simulink model "IEEE30_case"  (R2024b)
settings: Solver=FixedStepAuto  StartTime=0  StopTime=5  FixedStep=1e-7  RelTol=1e-3
values from neighbouring files (symbols this model uses):
  GFL_DFIG_7_C_bus = 0.08    [IEEE30_case_parameters.m]
  GFL_DFIG_7_D_mutual = 2.500000e+3    (= 2500)    [IEEE30_case_parameters.m]
  GFL_DFIG_7_f0 = 60    [IEEE30_case_parameters.m]
  GFL_DFIG_7_gPLLi = 3200    [IEEE30_case_parameters.m]
  GFL_DFIG_7_gPLLp = 650    [IEEE30_case_parameters.m]
  GFL_DFIG_7_H_WT = 0.4    [IEEE30_case_parameters.m]
  GFL_DFIG_7_Hg = 0.8    [IEEE30_case_parameters.m]
  GFL_DFIG_7_Igq_ref = 0    [IEEE30_case_parameters.m]
  GFL_DFIG_7_Ird_ref = 704.45696    [IEEE30_case_parameters.m]
  GFL_DFIG_7_KI_V = -300000    [IEEE30_case_parameters.m]
  GFL_DFIG_7_KP_V = -1000    [IEEE30_case_parameters.m]
  GFL_DFIG_7_Ksh = 1.254300e+4    (= 12543)    [IEEE30_case_parameters.m]
  GFL_DFIG_7_Lg = 0.000483    [IEEE30_case_parameters.m]
  GFL_DFIG_7_Lm_pu = 4    [IEEE30_case_parameters.m]
  GFL_DFIG_7_N = 100    [IEEE30_case_parameters.m]
  GFL_DFIG_7_p = 2    [IEEE30_case_parameters.m]
  GFL_DFIG_7_Pitch = 0    [IEEE30_case_parameters.m]
  GFL_DFIG_7_R = 44    [IEEE30_case_parameters.m]
  GFL_DFIG_7_Rg = 2.000000e-5    (= 2e-05)    [IEEE30_case_parameters.m]
  GFL_DFIG_7_rho = 1.225    [IEEE30_case_parameters.m]
  GFL_DFIG_7_rPLLi = 4500    [IEEE30_case_parameters.m]
  GFL_DFIG_7_rPLLp = 620    [IEEE30_case_parameters.m]
  GFL_DFIG_7_Rs_pu = 0.011    [IEEE30_case_parameters.m]
  GFL_DFIG_7_Sbase = 2.000000e+6    (= 2000000)    [IEEE30_case_parameters.m]
  GFL_DFIG_7_ugq_ref = 0    [IEEE30_case_parameters.m]
  GFL_DFIG_7_usd_ref = 0    [IEEE30_case_parameters.m]
  GFL_DFIG_7_Vbase = 690    [IEEE30_case_parameters.m]
  GFL_DFIG_7_Vdc_ref = 1200    [IEEE30_case_parameters.m]
  GFL_DFIG_7_wind = 12    [IEEE30_case_parameters.m]
  GFL_DFIG_7_wm_ref = 518.184209    [IEEE30_case_parameters.m]
  SG_D_13_D = 0.01056    [IEEE30_case_parameters.m]
  SG_D_13_EnableSaturation = 0    [IEEE30_case_parameters.m]
  SG_D_13_f0 = 60    [IEEE30_case_parameters.m]
  SG_D_13_H = 7.5    [IEEE30_case_parameters.m]
  SG_D_13_K_A = 20    [IEEE30_case_parameters.m]
  SG_D_13_K_E = 1.000000e+1    (= 10)    [IEEE30_case_parameters.m]
  SG_D_13_K_F = 2.363    [IEEE30_case_parameters.m]
  SG_D_13_K_s = 0.5    [IEEE30_case_parameters.m]
  SG_D_13_R_a = 0.001088    [IEEE30_case_parameters.m]
  SG_D_13_S_A = 1    [IEEE30_case_parameters.m]
  SG_D_13_S_B = 0.103    [IEEE30_case_parameters.m]
  SG_D_13_S_N = 10.659857    [IEEE30_case_parameters.m]
  SG_D_13_SpeedPara = 200    [IEEE30_case_parameters.m]
  SG_D_13_T_0 = 0.370163    [IEEE30_case_parameters.m]
  SG_D_13_T_1 = 0.3    [IEEE30_case_parameters.m]
  SG_D_13_T_2 = 0.05    [IEEE30_case_parameters.m]
  SG_D_13_T_3 = 0.02    [IEEE30_case_parameters.m]
  SG_D_13_T_4 = 0.005    [IEEE30_case_parameters.m]
  SG_D_13_T_A = 0.02    [IEEE30_case_parameters.m]
  SG_D_13_T_dd = 8.000000e+0    (= 8)    [IEEE30_case_parameters.m]
  SG_D_13_T_ddd = 0.04    [IEEE30_case_parameters.m]
  SG_D_13_T_E = 0.314    [IEEE30_case_parameters.m]
  SG_D_13_T_F = 0.35    [IEEE30_case_parameters.m]
  SG_D_13_T_qd = 0.8    [IEEE30_case_parameters.m]
  SG_D_13_T_qdd = 0.02    [IEEE30_case_parameters.m]
  SG_D_13_T_speed = 0.1    [IEEE30_case_parameters.m]
  SG_D_13_T_w = 0.5    [IEEE30_case_parameters.m]
  SG_D_13_V_ref = 1.696619    [IEEE30_case_parameters.m]
  SG_D_13_w_ref = 376.991118    [IEEE30_case_parameters.m]
  SG_D_13_x_d = 1.9    [IEEE30_case_parameters.m]
  SG_D_13_x_dd = 0.302    [IEEE30_case_parameters.m]
  SG_D_13_x_ddd = 0.204    [IEEE30_case_parameters.m]
  SG_D_13_x_l = 0.05    [IEEE30_case_parameters.m]
  SG_D_13_x_q = 1.3    [IEEE30_case_parameters.m]
  SG_D_13_x_qd = 0.5    [IEEE30_case_parameters.m]
  SG_D_13_x_qdd = 0.3    [IEEE30_case_parameters.m]
  SG_D_1_D = 0.01056    [IEEE30_case_parameters.m]
  SG_D_1_EnableSaturation = 0    [IEEE30_case_parameters.m]
  SG_D_1_f0 = 60    [IEEE30_case_parameters.m]
  SG_D_1_H = 7.5    [IEEE30_case_parameters.m]
  SG_D_1_K_A = 20    [IEEE30_case_parameters.m]
  SG_D_1_K_E = 1.000000e+1    (= 10)    [IEEE30_case_parameters.m]
  SG_D_1_K_F = 2.363    [IEEE30_case_parameters.m]
  SG_D_1_K_s = 0.5    [IEEE30_case_parameters.m]
  SG_D_1_R_a = 0.001088    [IEEE30_case_parameters.m]
  SG_D_1_S_A = 1    [IEEE30_case_parameters.m]
  SG_D_1_S_B = 0.103    [IEEE30_case_parameters.m]
  SG_D_1_S_N = 10.659857    [IEEE30_case_parameters.m]
  SG_D_1_SpeedPara = 200    [IEEE30_case_parameters.m]
  SG_D_1_T_0 = 0.259812    [IEEE30_case_parameters.m]
  SG_D_1_T_1 = 0.3    [IEEE30_case_parameters.m]
  SG_D_1_T_2 = 0.05    [IEEE30_case_parameters.m]
  SG_D_1_T_3 = 0.02    [IEEE30_case_parameters.m]
  SG_D_1_T_4 = 0.005    [IEEE30_case_parameters.m]
  SG_D_1_T_A = 0.02    [IEEE30_case_parameters.m]
  SG_D_1_T_dd = 8.000000e+0    (= 8)    [IEEE30_case_parameters.m]
  SG_D_1_T_ddd = 0.04    [IEEE30_case_parameters.m]
  SG_D_1_T_E = 0.314    [IEEE30_case_parameters.m]
  SG_D_1_T_F = 0.35    [IEEE30_case_parameters.m]
  SG_D_1_T_qd = 0.8    [IEEE30_case_parameters.m]
  SG_D_1_T_qdd = 0.02    [IEEE30_case_parameters.m]
  SG_D_1_T_speed = 0.1    [IEEE30_case_parameters.m]
  SG_D_1_T_w = 0.5    [IEEE30_case_parameters.m]
  SG_D_1_V_ref = 1.544107    [IEEE30_case_parameters.m]
  SG_D_1_w_ref = 376.991118    [IEEE30_case_parameters.m]
  SG_D_1_x_d = 1.9    [IEEE30_case_parameters.m]
  SG_D_1_x_dd = 0.302    [IEEE30_case_parameters.m]
  SG_D_1_x_ddd = 0.204    [IEEE30_case_parameters.m]
  SG_D_1_x_l = 0.05    [IEEE30_case_parameters.m]
  SG_D_1_x_q = 1.3    [IEEE30_case_parameters.m]
  SG_D_1_x_qd = 0.5    [IEEE30_case_parameters.m]
  SG_D_1_x_qdd = 0.3    [IEEE30_case_parameters.m]
  SG_D_22_D = 0.01056    [IEEE30_case_parameters.m]
  SG_D_22_EnableSaturation = 0    [IEEE30_case_parameters.m]
  SG_D_22_f0 = 60    [IEEE30_case_parameters.m]
  SG_D_22_H = 7.5    [IEEE30_case_parameters.m]
  SG_D_22_K_A = 20    [IEEE30_case_parameters.m]
  SG_D_22_K_E = 1.000000e+1    (= 10)    [IEEE30_case_parameters.m]
  SG_D_22_K_F = 2.363    [IEEE30_case_parameters.m]
  SG_D_22_K_s = 0.5    [IEEE30_case_parameters.m]
  SG_D_22_R_a = 0.001088    [IEEE30_case_parameters.m]
  SG_D_22_S_A = 1    [IEEE30_case_parameters.m]
  SG_D_22_S_B = 0.103    [IEEE30_case_parameters.m]
  SG_D_22_S_N = 10.659857    [IEEE30_case_parameters.m]
  SG_D_22_SpeedPara = 200    [IEEE30_case_parameters.m]
  SG_D_22_T_0 = 0.216121    [IEEE30_case_parameters.m]
  SG_D_22_T_1 = 0.3    [IEEE30_case_parameters.m]
  SG_D_22_T_2 = 0.05    [IEEE30_case_parameters.m]
  SG_D_22_T_3 = 0.02    [IEEE30_case_parameters.m]
  SG_D_22_T_4 = 0.005    [IEEE30_case_parameters.m]
  ... (+126 more)
(part 24 of 27)

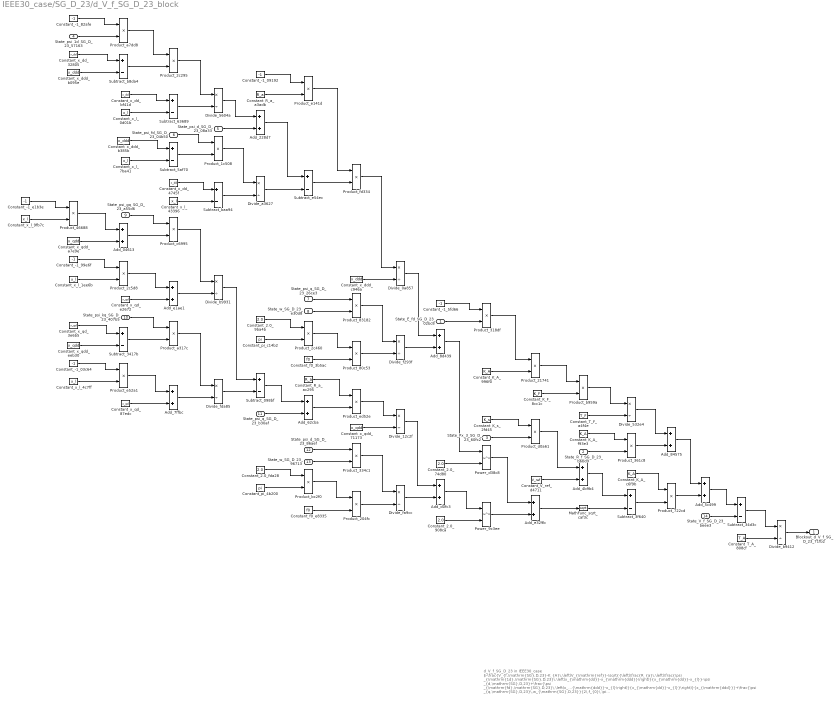
== system IEEE30_case/SG_D_23/d_V_f_SG_D_23_block ==
  note: d_V_f_SG_D_23 in IEEE30_case
      | $-\frac{V_{f,\mathrm{SG},D,23}-K_{A}\,\left(V_{\mathrm{ref}}-\sqrt{{\left(\frac{R_{a}\,\left(\frac{\psi _{\mathrm{1d},\mathrm{SG},D,23}\,\left(x_{\mathrm{dd}}-x_{\mathrm{ddd}}\right)}{x_{\mathrm{dd}}-x_{l}}-\psi _{d,\mathrm{SG},D,23}+\frac{\psi _{\mathrm{fd},\mathrm{SG},D,23}\,\left(x_{\mathrm{ddd}}-x_{l}\right)}{x_{\mathrm{dd}}-x_{l}}\right)}{x_{\mathrm{ddd}}}+\frac{\psi _{q,\mathrm{SG},D,23}\,w_{\mathrm{SG},D,23}}{2\,f_{0}\,\pi }\right)}^2+{\left(\frac{R_{a}\,\left(\psi _{q,\mathrm{SG},D,23}+\frac{\psi _{\mathrm{gq},\mathrm{SG},D,23}\,\left(x_{l}-x_{\mathrm{qdd}}\right)}{x_{l}-x_{\mathrm{qd}}}+\frac{\psi _{\mathrm{kq},\mathrm{SG},D,23}\,\left(x_{\mathrm{qd}}-x_{\mathrm{qdd}}\right)}{x_{l}-x_{\mathrm{qd}}}\right)}{x_{\mathrm{qdd}}}+\frac{\psi _{d,\mathrm{SG},D,23}\,w_{\mathrm{SG},D,23}}{2\,f_{0}\,\pi }\right)}^2}+K_{s}\,\mathrm{Px}_{3,\mathrm{SG},D,23}\right)-K_{A}\,R_{f,\mathrm{SG},D,23}+\frac{E_{\mathrm{fd},\mathrm{SG},D,23}\,K_{A}\,K_{F}}{T_{F}}}{T_{A}}$
      | Automatically generated on 2025-11-01 18:37:37 .
  State_E_fd_SG_D_23_02bc8 : Inport
  State_R_f_SG_D_23_b6bd9 : Inport  Port=2
  State_Px_3_SG_D_23_60fc2 : Inport  Port=3
  State_psi_1d_SG_D_23_57163 : Inport  Port=4
  State_psi_d_SG_D_23_08a33 : Inport  Port=5
  State_psi_fd_SG_D_23_04b50 : Inport  Port=6
  State_psi_q_SG_D_23_26ce3 : Inport  Port=7
  State_w_SG_D_23_e30d8 : Inport  Port=8
  State_psi_gq_SG_D_23_a55d6 : Inport  Port=9
  State_psi_kq_SG_D_23_407b5 : Inport  Port=10
  State_psi_q_SG_D_23_b30af : Inport  Port=11
  State_psi_d_SG_D_23_86aef : Inport  Port=12
  State_w_SG_D_23_96713 : Inport  Port=13
  State_V_f_SG_D_23_beee3 : Inport  Port=14
  Add_04613 : Sum
  Add_228d7 : Sum
  Add_4b9b4 : Sum
  Add_5c499 : Sum
  Add_62cba : Sum
  Add_7ffbc : Sum
  Add_84575 : Sum
  Add_8d439 : Sum
  Add_d0fc3 : Sum
  Add_e1ae1 : Sum
  Add_e329b : Sum
  Constant_-1_03c64 : Constant  Value=-1
  Constant_-1_09192 : Constant  Value=-1
  Constant_-1_5fd66 : Constant  Value=-1
  Constant_-1_82afe : Constant  Value=-1
  Constant_-1_99e6f : Constant  Value=-1
  Constant_-1_e1b3e : Constant  Value=-1
  Constant_2.0_74d80 : Constant  Value=2.0
  Constant_2.0_908ca : Constant  Value=2.0
  Constant_2.0_9ba4b : Constant  Value=2.0
  Constant_2.0_fda28 : Constant  Value=2.0
  Constant_K_A_996f0 : Constant  Value=K_A
  Constant_K_A_c6f9b : Constant  Value=K_A
  Constant_K_A_f93e3 : Constant  Value=K_A
  Constant_K_F_8cc1c : Constant  Value=K_F
  Constant_K_s_2fd45 : Constant  Value=K_s
  Constant_R_a_a3adb : Constant  Value=R_a
  Constant_R_a_ac295 : Constant  Value=R_a
  Constant_T_A_808cf : Constant  Value=T_A
  Constant_T_F_a4f4e : Constant  Value=T_F
  Constant_V_ref_d4711 : Constant  Value=V_ref
  Constant_f0_3b5ac : Constant  Value=f0
  Constant_f0_e8335 : Constant  Value=f0
  Constant_pi_4b200 : Constant  Value=pi
  Constant_pi_c14b2 : Constant  Value=pi
  Constant_x_dd_32805 : Constant  Value=x_dd
  Constant_x_dd_4745f : Constant  Value=x_dd
  Constant_x_dd_bf41d : Constant  Value=x_dd
  Constant_x_ddd_b095e : Constant  Value=x_ddd
  Constant_x_ddd_b385b : Constant  Value=x_ddd
  Constant_x_ddd_c946a : Constant  Value=x_ddd
  Constant_x_l_0d01b : Constant  Value=x_l
  Constant_x_l_1ee6b : Constant  Value=x_l
  Constant_x_l_43396 : Constant  Value=x_l
  Constant_x_l_4c7ff : Constant  Value=x_l
  Constant_x_l_7ba41 : Constant  Value=x_l
  Constant_x_l_9fb7c : Constant  Value=x_l
  Constant_x_qd_3e6b5 : Constant  Value=x_qd
  Constant_x_qd_87edc : Constant  Value=x_qd
  Constant_x_qd_e2672 : Constant  Value=x_qd
  Constant_x_qdd_71173 : Constant  Value=x_qdd
  Constant_x_qdd_a7e9e : Constant  Value=x_qdd
  Constant_x_qdd_eeb30 : Constant  Value=x_qdd
  Divide_0a857 : Product  Inputs=*/
  Divide_12c2f : Product  Inputs=*/
  Divide_532e4 : Product  Inputs=*/
  Divide_5604a : Product  Inputs=*/
  Divide_a3627 : Product  Inputs=*/
  Divide_b9412 : Product  Inputs=*/
  Divide_b9931 : Product  Inputs=*/
  Divide_f293f : Product  Inputs=*/
  Divide_fa9cc : Product  Inputs=*/
  Divide_fda85 : Product  Inputs=*/
  MathFunc_sqrt_caf3c : Sqrt
  Power_9c3ee : Math  Operator=pow
  Power_d38c8 : Math  Operator=pow
  Product_1c508 : Product
  Product_204fc : Product
  Product_21741 : Product
  Product_2c295 : Product
  Product_2c460 : Product
  Product_2c5d8 : Product
  Product_318df : Product
  Product_334c1 : Product
  Product_361c8 : Product
  Product_46688 : Product
  Product_722cd : Product
  Product_80c53 : Product
  Product_83182 : Product
  Product_a317c : Product
  Product_a7dd8 : Product
  Product_b959a : Product
  Product_bc2f0 : Product
  Product_c6995 : Product
  Product_d0a61 : Product
  Product_e141d : Product
  Product_e52a1 : Product
  Product_ed52e : Product
  Product_fd334 : Product
  Subtract_098bf : Sum  Inputs=+-
  Subtract_3417b : Sum  Inputs=+-
  Subtract_34d3c : Sum  Inputs=+-
  Subtract_3f640 : Sum  Inputs=+-
  Subtract_5af70 : Sum  Inputs=+-
  Subtract_63689 : Sum  Inputs=+-
  Subtract_b8da4 : Sum  Inputs=+-
  Subtract_baa94 : Sum  Inputs=+-
  Subtract_e54ec : Sum  Inputs=+-
  Blockout_d_V_f_SG_D_23_71fb2 : Outport
  wires:
  Constant_-1_e1b3e/1 -> Product_46688/1
  Add_228d7/1 -> Subtract_e54ec/1
  Constant_x_l_9fb7c/1 -> Product_46688/2
  Constant_-1_82afe/1 -> Product_a7dd8/1
  Product_2c5d8/1 -> Add_e1ae1/1
  State_psi_1d_SG_D_23_57163/1 -> Product_a7dd8/2
  Constant_x_dd_32805/1 -> Subtract_b8da4/1
  Divide_5604a/1 -> Add_228d7/1
  Constant_x_qdd_a7e9e/1 -> Add_04613/2
  Subtract_3417b/1 -> Product_a317c/2
  Constant_x_ddd_b095e/1 -> Subtract_b8da4/2
  Product_46688/1 -> Add_04613/1
  Constant_-1_99e6f/1 -> Product_2c5d8/1
  State_psi_d_SG_D_23_86aef/1 -> Product_334c1/1
  Constant_x_l_1ee6b/1 -> Product_2c5d8/2
  State_psi_d_SG_D_23_08a33/1 -> Add_228d7/2
  Divide_0a857/1 -> Add_8d439/1
  Constant_x_qd_3e6b5/1 -> Subtract_3417b/1
  Constant_x_qdd_eeb30/1 -> Subtract_3417b/2
  Constant_-1_03c64/1 -> Product_e52a1/1
  Constant_x_l_4c7ff/1 -> Product_e52a1/2
  Constant_R_a_a3adb/1 -> Product_e141d/2
  Product_a7dd8/1 -> Product_2c295/1
  Subtract_b8da4/1 -> Product_2c295/2
  Constant_2.0_fda28/1 -> Product_bc2f0/1
  Constant_x_dd_bf41d/1 -> Subtract_63689/1
  Product_e141d/1 -> Product_fd334/1
  Add_7ffbc/1 -> Divide_fda85/2
  Constant_pi_4b200/1 -> Product_bc2f0/2
  Constant_x_l_0d01b/1 -> Subtract_63689/2
  Constant_f0_3b5ac/1 -> Product_80c53/2
  Constant_x_ddd_b385b/1 -> Subtract_5af70/1
  Constant_x_l_7ba41/1 -> Subtract_5af70/2
  State_psi_gq_SG_D_23_a55d6/1 -> Product_c6995/1
  Constant_K_A_f93e3/1 -> Product_361c8/1
  State_w_SG_D_23_e30d8/1 -> Product_83182/2
  Add_04613/1 -> Product_c6995/2
  Product_2c295/1 -> Divide_5604a/1
  Constant_x_qd_e2672/1 -> Add_e1ae1/2
  State_w_SG_D_23_96713/1 -> Product_334c1/2
  State_psi_kq_SG_D_23_407b5/1 -> Product_a317c/1
  Constant_-1_09192/1 -> Product_e141d/1
  Constant_f0_e8335/1 -> Product_204fc/2
  Product_e52a1/1 -> Add_7ffbc/1
  Constant_x_qd_87edc/1 -> Add_7ffbc/2
  Add_e1ae1/1 -> Divide_b9931/2
  Subtract_63689/1 -> Divide_5604a/2
  State_psi_fd_SG_D_23_04b50/1 -> Product_1c508/1
  Constant_pi_c14b2/1 -> Product_2c460/2
  Subtract_5af70/1 -> Product_1c508/2
  Constant_x_dd_4745f/1 -> Subtract_baa94/1
  Constant_x_l_43396/1 -> Subtract_baa94/2
  Product_c6995/1 -> Divide_b9931/1
  Product_a317c/1 -> Divide_fda85/1
  Product_1c508/1 -> Divide_a3627/1
  Subtract_baa94/1 -> Divide_a3627/2
  Divide_b9931/1 -> Subtract_098bf/1
  Divide_fda85/1 -> Subtract_098bf/2
  Divide_a3627/1 -> Subtract_e54ec/2
  Constant_2.0_9ba4b/1 -> Product_2c460/1
  Subtract_098bf/1 -> Add_62cba/1
  State_psi_q_SG_D_23_b30af/1 -> Add_62cba/2
  Subtract_e54ec/1 -> Product_fd334/2
  State_psi_q_SG_D_23_26ce3/1 -> Product_83182/1
  Product_2c460/1 -> Product_80c53/1
  Constant_R_a_ac295/1 -> Product_ed52e/1
  Add_62cba/1 -> Product_ed52e/2
  Product_bc2f0/1 -> Product_204fc/1
  Product_fd334/1 -> Divide_0a857/1
  Constant_x_ddd_c946a/1 -> Divide_0a857/2
  Product_83182/1 -> Divide_f293f/1
  Product_80c53/1 -> Divide_f293f/2
  Product_21741/1 -> Product_b959a/1
  Product_ed52e/1 -> Divide_12c2f/1
  Constant_x_qdd_71173/1 -> Divide_12c2f/2
  Product_334c1/1 -> Divide_fa9cc/1
  Product_204fc/1 -> Divide_fa9cc/2
  Divide_f293f/1 -> Add_8d439/2
  Product_b959a/1 -> Divide_532e4/1
  Divide_12c2f/1 -> Add_d0fc3/1
  Divide_fa9cc/1 -> Add_d0fc3/2
  Constant_-1_5fd66/1 -> Product_318df/1
  State_E_fd_SG_D_23_02bc8/1 -> Product_318df/2
  Add_8d439/1 -> Power_d38c8/1
  Constant_2.0_74d80/1 -> Power_d38c8/2
  Add_d0fc3/1 -> Power_9c3ee/1
  Constant_2.0_908ca/1 -> Power_9c3ee/2
  Product_318df/1 -> Product_21741/1
  Constant_K_A_996f0/1 -> Product_21741/2
  Constant_K_s_2fd45/1 -> Product_d0a61/1
  State_Px_3_SG_D_23_60fc2/1 -> Product_d0a61/2
  Power_d38c8/1 -> Add_e329b/1
  Add_84575/1 -> Add_5c499/1
  Power_9c3ee/1 -> Add_e329b/2
  Constant_K_F_8cc1c/1 -> Product_b959a/2
  Product_d0a61/1 -> Add_4b9b4/1
  Constant_V_ref_d4711/1 -> Add_4b9b4/2
  Add_e329b/1 -> MathFunc_sqrt_caf3c/1
  Constant_T_F_a4f4e/1 -> Divide_532e4/2
  State_R_f_SG_D_23_b6bd9/1 -> Product_361c8/2
  Add_4b9b4/1 -> Subtract_3f640/1
  MathFunc_sqrt_caf3c/1 -> Subtract_3f640/2
  Divide_532e4/1 -> Add_84575/1
  Product_361c8/1 -> Add_84575/2
  Constant_K_A_c6f9b/1 -> Product_722cd/1
  Subtract_3f640/1 -> Product_722cd/2
  Product_722cd/1 -> Add_5c499/2
  Add_5c499/1 -> Subtract_34d3c/1
  State_V_f_SG_D_23_beee3/1 -> Subtract_34d3c/2
  Subtract_34d3c/1 -> Divide_b9412/1
  Constant_T_A_808cf/1 -> Divide_b9412/2
  Divide_b9412/1 -> Blockout_d_V_f_SG_D_23_71fb2/1

== system IEEE30_case/SG_D_23/d_psi_1d_SG_D_23_block ==
  note: d_psi_1d_SG_D_23 in IEEE30_case
      | $-\frac{\psi _{\mathrm{1d},\mathrm{SG},D,23}-\psi _{\mathrm{fd},\mathrm{SG},D,23}+\frac{\left(x_{\mathrm{dd}}-x_{l}\right)\,\left(\frac{\psi _{\mathrm{1d},\mathrm{SG},D,23}\,\left(x_{\mathrm{dd}}-x_{\mathrm{ddd}}\right)}{x_{\mathrm{dd}}-x_{l}}-\psi _{d,\mathrm{SG},D,23}+\frac{\psi _{\mathrm{fd},\mathrm{SG},D,23}\,\left(x_{\mathrm{ddd}}-x_{l}\right)}{x_{\mathrm{dd}}-x_{l}}\right)}{x_{\mathrm{ddd}}}}{T_{\mathrm{ddd}}}$
      | Automatically generated on 2025-11-01 18:37:11 .
  State_psi_1d_SG_D_23_f9ad5 : Inport
  State_psi_fd_SG_D_23_0adb9 : Inport  Port=2
  State_psi_1d_SG_D_23_5015b : Inport  Port=3
  State_psi_d_SG_D_23_22f26 : Inport  Port=4
  State_psi_fd_SG_D_23_ec5fd : Inport  Port=5
  Add_56ba0 : Sum
  Add_88951 : Sum
  Add_9af81 : Sum
  Constant_-1_6d8e7 : Constant  Value=-1
  Constant_-1_81748 : Constant  Value=-1
  Constant_T_ddd_a7ba2 : Constant  Value=T_ddd
  Constant_x_dd_7d3aa : Constant  Value=x_dd
  Constant_x_dd_a16d9 : Constant  Value=x_dd
  Constant_x_dd_cf2ad : Constant  Value=x_dd
  Constant_x_dd_edf45 : Constant  Value=x_dd
  Constant_x_ddd_8324c : Constant  Value=x_ddd
  Constant_x_ddd_b932a : Constant  Value=x_ddd
  Constant_x_ddd_d8375 : Constant  Value=x_ddd
  Constant_x_l_201dc : Constant  Value=x_l
  Constant_x_l_34716 : Constant  Value=x_l
  Constant_x_l_5fce1 : Constant  Value=x_l
  Constant_x_l_b924b : Constant  Value=x_l
  Divide_17a42 : Product  Inputs=*/
  Divide_37bc4 : Product  Inputs=*/
  Divide_469be : Product  Inputs=*/
  Divide_d9984 : Product  Inputs=*/
  Product_2d7ae : Product
  Product_86568 : Product
  Product_9e087 : Product
  Product_afbd6 : Product
  Product_d6b36 : Product
  Subtract_2aa7c : Sum  Inputs=+-
  Subtract_6fe59 : Sum  Inputs=+-
  Subtract_9814b : Sum  Inputs=+-
  Subtract_a17ec : Sum  Inputs=+-
  Subtract_ba284 : Sum  Inputs=+-
  Subtract_c73aa : Sum  Inputs=+-
  Blockout_d_psi_1d_SG_D_23_c2996 : Outport
  wires:
  Constant_-1_6d8e7/1 -> Product_86568/1
  State_psi_1d_SG_D_23_5015b/1 -> Product_86568/2
  Constant_x_ddd_8324c/1 -> Subtract_2aa7c/1
  Constant_x_dd_7d3aa/1 -> Subtract_ba284/1
  Constant_x_ddd_d8375/1 -> Subtract_ba284/2
  Product_86568/1 -> Product_d6b36/1
  Subtract_ba284/1 -> Product_d6b36/2
  State_psi_d_SG_D_23_22f26/1 -> Add_88951/2
  Constant_x_dd_edf45/1 -> Subtract_c73aa/1
  Constant_x_l_b924b/1 -> Subtract_c73aa/2
  Add_9af81/1 -> Divide_37bc4/1
  Add_88951/1 -> Subtract_a17ec/1
  Constant_x_l_34716/1 -> Subtract_2aa7c/2
  State_psi_fd_SG_D_23_0adb9/1 -> Add_56ba0/2
  Product_d6b36/1 -> Divide_17a42/1
  Subtract_c73aa/1 -> Divide_17a42/2
  State_psi_fd_SG_D_23_ec5fd/1 -> Product_2d7ae/1
  Constant_x_l_5fce1/1 -> Subtract_6fe59/2
  Subtract_2aa7c/1 -> Product_2d7ae/2
  Constant_x_dd_cf2ad/1 -> Subtract_9814b/1
  Constant_x_l_201dc/1 -> Subtract_9814b/2
  Divide_17a42/1 -> Add_88951/1
  Product_2d7ae/1 -> Divide_469be/1
  Subtract_9814b/1 -> Divide_469be/2
  Constant_x_dd_a16d9/1 -> Subtract_6fe59/1
  Divide_469be/1 -> Subtract_a17ec/2
  Constant_-1_81748/1 -> Product_afbd6/1
  State_psi_1d_SG_D_23_f9ad5/1 -> Product_afbd6/2
  Subtract_6fe59/1 -> Product_9e087/1
  Subtract_a17ec/1 -> Product_9e087/2
  Product_afbd6/1 -> Add_56ba0/1
  Product_9e087/1 -> Divide_d9984/1
  Constant_x_ddd_b932a/1 -> Divide_d9984/2
  Add_56ba0/1 -> Add_9af81/1
  Divide_d9984/1 -> Add_9af81/2
  Constant_T_ddd_a7ba2/1 -> Divide_37bc4/2
  Divide_37bc4/1 -> Blockout_d_psi_1d_SG_D_23_c2996/1

== system IEEE30_case/SG_D_23/d_psi_d_SG_D_23_block ==
  note: d_psi_d_SG_D_23 in IEEE30_case
      | $2\,\pi \,f_{0}\,\left(v_{d,\mathrm{SG},D,23}\,\sin\left(\theta _{\mathrm{SG},D,23}\right)-v_{q,\mathrm{SG},D,23}\,\cos\left(\theta _{\mathrm{SG},D,23}\right)+\frac{R_{a}\,\left(\frac{\psi _{\mathrm{1d},\mathrm{SG},D,23}\,\left(x_{\mathrm{dd}}-x_{\mathrm{ddd}}\right)}{x_{\mathrm{dd}}-x_{l}}-\psi _{d,\mathrm{SG},D,23}+\frac{\psi _{\mathrm{fd},\mathrm{SG},D,23}\,\left(x_{\mathrm{ddd}}-x_{l}\right)}{x_{\mathrm{dd}}-x_{l}}\right)}{x_{\mathrm{ddd}}}+\frac{\psi _{q,\mathrm{SG},D,23}\,w_{\mathrm{SG},D,23}}{2\,f_{0}\,\pi }\right)$
      | Automatically generated on 2025-11-01 18:36:59 .
  State_psi_1d_SG_D_23_8965f : Inport
  State_psi_d_SG_D_23_016fe : Inport  Port=2
  State_psi_fd_SG_D_23_f3d1f : Inport  Port=3
  Input_v_d_SG_D_23_9e347 : Inport  Port=4
  State_theta_SG_D_23_2ec18 : Inport  Port=5
  Input_v_q_SG_D_23_ae17a : Inport  Port=6
  State_theta_SG_D_23_794b5 : Inport  Port=7
  State_psi_q_SG_D_23_bc7c3 : Inport  Port=8
  State_w_SG_D_23_6d242 : Inport  Port=9
  Add_d73dc : Sum
  Add_ea58b : Sum
  Constant_-1_12cc8 : Constant  Value=-1
  Constant_-2.0_fa6bb : Constant  Value=-2.0
  Constant_2.0_bdbff : Constant  Value=2.0
  Constant_R_a_3ad34 : Constant  Value=R_a
  Constant_f0_d5693 : Constant  Value=f0
  Constant_f0_f51c1 : Constant  Value=f0
  Constant_pi_649aa : Constant  Value=pi
  Constant_pi_fa739 : Constant  Value=pi
  Constant_x_dd_172d9 : Constant  Value=x_dd
  Constant_x_dd_52223 : Constant  Value=x_dd
  Constant_x_dd_c8000 : Constant  Value=x_dd
  Constant_x_ddd_1f572 : Constant  Value=x_ddd
  Constant_x_ddd_7d6d0 : Constant  Value=x_ddd
  Constant_x_ddd_ee30d : Constant  Value=x_ddd
  Constant_x_l_54e71 : Constant  Value=x_l
  Constant_x_l_639de : Constant  Value=x_l
  Constant_x_l_b39fb : Constant  Value=x_l
  Divide_513f6 : Product  Inputs=*/
  Divide_6520c : Product  Inputs=*/
  Divide_8ac7a : Product  Inputs=*/
  Divide_e7c9b : Product  Inputs=*/
  MathFunc_cos_10b2b : Trigonometry  Operator=cos
  MathFunc_sin_15f05 : Trigonometry
  Product_2a9f7 : Product
  Product_31118 : Product
  Product_38c7b : Product
  Product_5e2c6 : Product
  Product_62de7 : Product
  Product_737bc : Product
  Product_7e675 : Product
  Product_98a77 : Product
  Product_b1903 : Product
  Product_bad50 : Product
  Product_ce148 : Product
  Product_ee1e8 : Product
  Subtract_18b3f : Sum  Inputs=+-
  Subtract_1f850 : Sum  Inputs=+-
  Subtract_2847e : Sum  Inputs=+-
  Subtract_314f8 : Sum  Inputs=+-
  Subtract_971ca : Sum  Inputs=+-
  Subtract_d4bdb : Sum  Inputs=+-
  Subtract_de438 : Sum  Inputs=+-
  Blockout_d_psi_d_SG_D_23_781f9 : Outport
  wires:
  Constant_-1_12cc8/1 -> Product_ee1e8/1
  Product_ee1e8/1 -> Product_bad50/1
  Constant_x_dd_52223/1 -> Subtract_d4bdb/1
  Subtract_d4bdb/1 -> Product_bad50/2
  State_psi_1d_SG_D_23_8965f/1 -> Product_ee1e8/2
  Product_62de7/1 -> Divide_6520c/1
  Constant_x_ddd_7d6d0/1 -> Subtract_d4bdb/2
  Subtract_de438/1 -> Divide_8ac7a/2
  Constant_x_dd_c8000/1 -> Subtract_de438/1
  Constant_x_l_54e71/1 -> Subtract_de438/2
  State_w_SG_D_23_6d242/1 -> Product_5e2c6/2
  Constant_x_ddd_1f572/1 -> Subtract_18b3f/1
  Constant_x_l_639de/1 -> Subtract_18b3f/2
  Product_bad50/1 -> Divide_8ac7a/1
  State_psi_fd_SG_D_23_f3d1f/1 -> Product_2a9f7/1
  Product_737bc/1 -> Product_b1903/1
  Subtract_18b3f/1 -> Product_2a9f7/2
  Constant_x_dd_172d9/1 -> Subtract_314f8/1
  MathFunc_cos_10b2b/1 -> Product_38c7b/2
  State_theta_SG_D_23_794b5/1 -> MathFunc_cos_10b2b/1
  Constant_x_l_b39fb/1 -> Subtract_314f8/2
  Divide_8ac7a/1 -> Add_d73dc/1
  Subtract_1f850/1 -> Product_b1903/2
  State_psi_d_SG_D_23_016fe/1 -> Add_d73dc/2
  Product_2a9f7/1 -> Divide_513f6/1
  Subtract_314f8/1 -> Divide_513f6/2
  Add_d73dc/1 -> Subtract_2847e/1
  Constant_pi_fa739/1 -> Product_98a77/2
  Divide_513f6/1 -> Subtract_2847e/2
  Constant_R_a_3ad34/1 -> Product_62de7/1
  Subtract_2847e/1 -> Product_62de7/2
  Constant_f0_d5693/1 -> Product_31118/2
  State_theta_SG_D_23_2ec18/1 -> MathFunc_sin_15f05/1
  Constant_x_ddd_ee30d/1 -> Divide_6520c/2
  Product_ce148/1 -> Subtract_971ca/2
  Input_v_d_SG_D_23_9e347/1 -> Product_ce148/1
  MathFunc_sin_15f05/1 -> Product_ce148/2
  Product_7e675/1 -> Product_31118/1
  Constant_2.0_bdbff/1 -> Product_7e675/1
  Input_v_q_SG_D_23_ae17a/1 -> Product_38c7b/1
  Constant_pi_649aa/1 -> Product_7e675/2
  Divide_6520c/1 -> Subtract_971ca/1
  Product_b1903/1 -> Blockout_d_psi_d_SG_D_23_781f9/1
  Product_5e2c6/1 -> Divide_e7c9b/1
  State_psi_q_SG_D_23_bc7c3/1 -> Product_5e2c6/1
  Constant_-2.0_fa6bb/1 -> Product_98a77/1
  Subtract_971ca/1 -> Add_ea58b/1
  Product_38c7b/1 -> Add_ea58b/2
  Product_31118/1 -> Divide_e7c9b/2
  Product_98a77/1 -> Product_737bc/1
  Constant_f0_f51c1/1 -> Product_737bc/2
  Add_ea58b/1 -> Subtract_1f850/1
  Divide_e7c9b/1 -> Subtract_1f850/2

== system IEEE30_case/SG_D_23/d_psi_fd_SG_D_23_block ==
  note: d_psi_fd_SG_D_23 in IEEE30_case
      | $-\frac{\psi _{\mathrm{fd},\mathrm{SG},D,23}-E_{\mathrm{fd},\mathrm{SG},D,23}+\left(x_{d}-x_{\mathrm{dd}}\right)\,\left(\frac{\frac{\psi _{\mathrm{1d},\mathrm{SG},D,23}\,\left(x_{\mathrm{dd}}-x_{\mathrm{ddd}}\right)}{x_{\mathrm{dd}}-x_{l}}-\psi _{d,\mathrm{SG},D,23}+\frac{\psi _{\mathrm{fd},\mathrm{SG},D,23}\,\left(x_{\mathrm{ddd}}-x_{l}\right)}{x_{\mathrm{dd}}-x_{l}}}{x_{\mathrm{ddd}}}-\frac{\left(x_{\mathrm{dd}}-x_{\mathrm{ddd}}\right)\,\left(\psi _{\mathrm{1d},\mathrm{SG},D,23}-\psi _{\mathrm{fd},\mathrm{SG},D,23}+\frac{\left(x_{\mathrm{dd}}-x_{l}\right)\,\left(\frac{\psi _{\mathrm{1d},\mathrm{SG},D,23}\,\left(x_{\mathrm{dd}}-x_{\mathrm{ddd}}\right)}{x_{\mathrm{dd}}-x_{l}}-\psi _{d,\mathrm{SG},D,23}+\frac{\psi _{\mathrm{fd},\mathrm{SG},D,23}\,\left(x_{\mathrm{ddd}}-x_{l}\right)}{x_{\mathrm{dd}}-x_{l}}\right)}{x_{\mathrm{ddd}}}\right)}{{\left(x_{\mathrm{dd}}-x_{l}\right)}^2}\right)}{T_{\mathrm{dd}}}$
      | Automatically generated on 2025-11-01 18:37:09 .
  State_E_fd_SG_D_23_28355 : Inport
  State_psi_fd_SG_D_23_a87ca : Inport  Port=2
  State_psi_1d_SG_D_23_a98e3 : Inport  Port=3
  State_psi_fd_SG_D_23_d0500 : Inport  Port=4
  State_psi_1d_SG_D_23_20435 : Inport  Port=5
  State_psi_d_SG_D_23_5a21e : Inport  Port=6
  State_psi_fd_SG_D_23_a8ac0 : Inport  Port=7
  State_psi_1d_SG_D_23_3e436 : Inport  Port=8
  State_psi_d_SG_D_23_78162 : Inport  Port=9
  State_psi_fd_SG_D_23_640f3 : Inport  Port=10
  Add_36fcd : Sum
  Add_a626a : Sum
  Constant_-1_040f4 : Constant  Value=-1
  Constant_-1_24d46 : Constant  Value=-1
  Constant_-1_8a775 : Constant  Value=-1
  Constant_2.0_a8a6a : Constant  Value=2.0
  Constant_T_dd_8e02f : Constant  Value=T_dd
  Constant_x_d_69503 : Constant  Value=x_d
  Constant_x_dd_0f43c : Constant  Value=x_dd
  Constant_x_dd_3049e : Constant  Value=x_dd
  Constant_x_dd_31422 : Constant  Value=x_dd
  Constant_x_dd_43abf : Constant  Value=x_dd
  Constant_x_dd_670c2 : Constant  Value=x_dd
  Constant_x_dd_8e1c3 : Constant  Value=x_dd
  Constant_x_dd_94288 : Constant  Value=x_dd
  Constant_x_dd_9ceae : Constant  Value=x_dd
  Constant_x_dd_b82f4 : Constant  Value=x_dd
  Constant_x_dd_c9942 : Constant  Value=x_dd
  Constant_x_ddd_22d37 : Constant  Value=x_ddd
  Constant_x_ddd_53380 : Constant  Value=x_ddd
  Constant_x_ddd_869dc : Constant  Value=x_ddd
  Constant_x_ddd_a63b3 : Constant  Value=x_ddd
  Constant_x_ddd_e3405 : Constant  Value=x_ddd
  Constant_x_ddd_eca09 : Constant  Value=x_ddd
  Constant_x_ddd_f476d : Constant  Value=x_ddd
  Constant_x_l_27032 : Constant  Value=x_l
  Constant_x_l_3c9e7 : Constant  Value=x_l
  Constant_x_l_4375b : Constant  Value=x_l
  Constant_x_l_65007 : Constant  Value=x_l
  Constant_x_l_8ced4 : Constant  Value=x_l
  Constant_x_l_9c65e : Constant  Value=x_l
  Constant_x_l_a40c3 : Constant  Value=x_l
  Constant_x_l_b2234 : Constant  Value=x_l
  Divide_69c83 : Product  Inputs=*/
  Divide_6bb0f : Product  Inputs=*/
  Divide_82107 : Product  Inputs=*/
  Divide_8f783 : Product  Inputs=*/
  Divide_b15cd : Product  Inputs=*/
  Divide_c21b3 : Product  Inputs=*/
  Divide_ccb9e : Product  Inputs=*/
  Divide_ebecf : Product  Inputs=*/
  Power_2f5cb : Math  Operator=pow
  Product_283a6 : Product
  Product_7c461 : Product
  Product_7dee2 : Product
  Product_8c666 : Product
  Product_8ec8a : Product
  Product_95aa3 : Product
  Product_a796e : Product
  Product_bf0be : Product
  Product_cd65d : Product
  Product_f8c61 : Product
  Subtract_10bf5 : Sum  Inputs=+-
  Subtract_4c941 : Sum  Inputs=+-
  Subtract_540da : Sum  Inputs=+-
  Subtract_602f9 : Sum  Inputs=+-
  Subtract_6a387 : Sum  Inputs=+-
  Subtract_723f7 : Sum  Inputs=+-
  Subtract_80fe0 : Sum  Inputs=+-
  Subtract_872fd : Sum  Inputs=+-
  Subtract_9e3fc : Sum  Inputs=+-
  Subtract_afd8f : Sum  Inputs=+-
  Subtract_bca89 : Sum  Inputs=+-
  Subtract_bf7f4 : Sum  Inputs=+-
  Subtract_cda79 : Sum  Inputs=+-
  Subtract_ce83f : Sum  Inputs=+-
  Subtract_ce99a : Sum  Inputs=+-
  Subtract_d5253 : Sum  Inputs=+-
  Subtract_d7a89 : Sum  Inputs=+-
  Subtract_ec96d : Sum  Inputs=+-
  Subtract_fb10c : Sum  Inputs=+-
  Blockout_d_psi_fd_SG_D_23_cc715 : Outport
  wires:
  Subtract_723f7/1 -> Product_283a6/1
  Constant_x_l_27032/1 -> Subtract_602f9/2
  Constant_-1_040f4/1 -> Product_8ec8a/1
  Constant_x_dd_31422/1 -> Subtract_602f9/1
  Product_7dee2/1 -> Divide_6bb0f/1
  State_psi_1d_SG_D_23_20435/1 -> Product_8ec8a/2
  Constant_x_dd_670c2/1 -> Subtract_d7a89/1
  Constant_x_dd_b82f4/1 -> Subtract_723f7/1
  Constant_x_ddd_22d37/1 -> Subtract_d7a89/2
  Product_8ec8a/1 -> Product_7dee2/1
  Subtract_d7a89/1 -> Product_7dee2/2
  Constant_x_ddd_53380/1 -> Subtract_4c941/1
  Constant_x_dd_c9942/1 -> Subtract_afd8f/1
  Constant_x_l_65007/1 -> Subtract_4c941/2
  Subtract_602f9/1 -> Divide_6bb0f/2
  Constant_x_l_4375b/1 -> Subtract_afd8f/2
  State_E_fd_SG_D_23_28355/1 -> Subtract_ce83f/1
  State_psi_fd_SG_D_23_a8ac0/1 -> Product_8c666/1
  Constant_x_ddd_f476d/1 -> Divide_ebecf/2
  Subtract_4c941/1 -> Product_8c666/2
  Divide_6bb0f/1 -> Add_36fcd/1
  Constant_x_dd_3049e/1 -> Subtract_bf7f4/1
  State_psi_d_SG_D_23_5a21e/1 -> Add_36fcd/2
  Product_8c666/1 -> Divide_82107/1
  Subtract_afd8f/1 -> Divide_82107/2
  Constant_x_l_8ced4/1 -> Subtract_723f7/2
  Add_36fcd/1 -> Subtract_bca89/1
  Divide_82107/1 -> Subtract_bca89/2
  Constant_-1_8a775/1 -> Product_cd65d/1
  Product_cd65d/1 -> Product_95aa3/1
  State_psi_1d_SG_D_23_3e436/1 -> Product_cd65d/2
  Constant_x_dd_94288/1 -> Subtract_10bf5/1
  Constant_x_ddd_a63b3/1 -> Subtract_10bf5/2
  Subtract_bca89/1 -> Product_283a6/2
  Subtract_10bf5/1 -> Product_95aa3/2
  Constant_2.0_a8a6a/1 -> Power_2f5cb/2
  Constant_x_l_9c65e/1 -> Subtract_bf7f4/2
  Constant_x_dd_9ceae/1 -> Subtract_ce99a/1
  Constant_x_l_3c9e7/1 -> Subtract_ce99a/2
  Product_a796e/1 -> Product_f8c61/1
  Subtract_d5253/1 -> Product_7c461/2
  Constant_x_ddd_eca09/1 -> Subtract_d5253/1
  Subtract_540da/1 -> Divide_8f783/2
  Subtract_6a387/1 -> Product_a796e/2
  Constant_x_dd_43abf/1 -> Subtract_540da/1
  Constant_x_l_b2234/1 -> Subtract_d5253/2
  Constant_x_dd_0f43c/1 -> Subtract_6a387/1
  Constant_x_l_a40c3/1 -> Subtract_540da/2
  Constant_x_ddd_869dc/1 -> Subtract_6a387/2
  State_psi_1d_SG_D_23_a98e3/1 -> Subtract_872fd/1
  State_psi_fd_SG_D_23_d0500/1 -> Subtract_872fd/2
  Product_283a6/1 -> Divide_ebecf/1
  Product_95aa3/1 -> Divide_ccb9e/1
  Subtract_ce99a/1 -> Divide_ccb9e/2
  Product_7c461/1 -> Divide_8f783/1
  State_psi_fd_SG_D_23_640f3/1 -> Product_7c461/1
  Constant_-1_24d46/1 -> Product_a796e/1
  Subtract_872fd/1 -> Subtract_ec96d/1
  Divide_ebecf/1 -> Subtract_ec96d/2
  Divide_ccb9e/1 -> Add_a626a/1
  State_psi_d_SG_D_23_78162/1 -> Add_a626a/2
  Subtract_ec96d/1 -> Product_f8c61/2
  Subtract_bf7f4/1 -> Power_2f5cb/1
  Add_a626a/1 -> Subtract_fb10c/1
  Divide_8f783/1 -> Subtract_fb10c/2
  Product_f8c61/1 -> Divide_69c83/1
  Power_2f5cb/1 -> Divide_69c83/2
  Subtract_fb10c/1 -> Divide_c21b3/1
  Constant_x_ddd_e3405/1 -> Divide_c21b3/2
  Constant_x_d_69503/1 -> Subtract_cda79/1
  Constant_x_dd_8e1c3/1 -> Subtract_cda79/2
  Divide_69c83/1 -> Subtract_9e3fc/1
  Divide_c21b3/1 -> Subtract_9e3fc/2
  State_psi_fd_SG_D_23_a87ca/1 -> Subtract_ce83f/2
  Subtract_cda79/1 -> Product_bf0be/1
  Subtract_9e3fc/1 -> Product_bf0be/2
  Subtract_ce83f/1 -> Subtract_80fe0/1
  Product_bf0be/1 -> Subtract_80fe0/2
  Subtract_80fe0/1 -> Divide_b15cd/1
  Constant_T_dd_8e02f/1 -> Divide_b15cd/2
  Divide_b15cd/1 -> Blockout_d_psi_fd_SG_D_23_cc715/1

== system IEEE30_case/SG_D_23/d_psi_gq_SG_D_23_block ==
  note: d_psi_gq_SG_D_23 in IEEE30_case
      | $-\frac{\psi _{\mathrm{gq},\mathrm{SG},D,23}+\left(x_{q}-x_{\mathrm{qd}}\right)\,\left(\frac{\psi _{q,\mathrm{SG},D,23}+\frac{\psi _{\mathrm{gq},\mathrm{SG},D,23}\,\left(x_{l}-x_{\mathrm{qdd}}\right)}{x_{l}-x_{\mathrm{qd}}}+\frac{\psi _{\mathrm{kq},\mathrm{SG},D,23}\,\left(x_{\mathrm{qd}}-x_{\mathrm{qdd}}\right)}{x_{l}-x_{\mathrm{qd}}}}{x_{\mathrm{qdd}}}+\frac{\left(x_{\mathrm{qd}}-x_{\mathrm{qdd}}\right)\,\left(\psi _{\mathrm{gq},\mathrm{SG},D,23}+\psi _{\mathrm{kq},\mathrm{SG},D,23}+\frac{\left(x_{l}-x_{\mathrm{qd}}\right)\,\left(\psi _{q,\mathrm{SG},D,23}+\frac{\psi _{\mathrm{gq},\mathrm{SG},D,23}\,\left(x_{l}-x_{\mathrm{qdd}}\right)}{x_{l}-x_{\mathrm{qd}}}+\frac{\psi _{\mathrm{kq},\mathrm{SG},D,23}\,\left(x_{\mathrm{qd}}-x_{\mathrm{qdd}}\right)}{x_{l}-x_{\mathrm{qd}}}\right)}{x_{\mathrm{qdd}}}\right)}{{\left(x_{l}-x_{\mathrm{qd}}\right)}^2}\right)}{T_{\mathrm{qd}}}$
      | Automatically generated on 2025-11-01 18:37:17 .
  State_psi_gq_SG_D_23_15800 : Inport
  State_psi_gq_SG_D_23_52211 : Inport  Port=2
  State_psi_kq_SG_D_23_2d830 : Inport  Port=3
  State_psi_gq_SG_D_23_9dcc3 : Inport  Port=4
  State_psi_kq_SG_D_23_b4351 : Inport  Port=5
  State_psi_q_SG_D_23_fd8a2 : Inport  Port=6
  State_psi_gq_SG_D_23_02c8f : Inport  Port=7
  State_psi_kq_SG_D_23_c86ae : Inport  Port=8
  State_psi_q_SG_D_23_a58a4 : Inport  Port=9
  Add_07245 : Sum
  Add_1b597 : Sum
  Add_22213 : Sum
  Add_32192 : Sum
  Add_5c235 : Sum
  Add_5d65c : Sum
  Add_66016 : Sum
  Add_6eda3 : Sum
  Add_81c60 : Sum
  Add_b1f47 : Sum
  Add_ce471 : Sum
  Add_d9c53 : Sum
  Constant_-1_21c54 : Constant  Value=-1
  Constant_-1_5ec91 : Constant  Value=-1
  Constant_-1_74396 : Constant  Value=-1
  Constant_-1_b270e : Constant  Value=-1
  Constant_-1_c60a9 : Constant  Value=-1
  Constant_-1_d9c78 : Constant  Value=-1
  Constant_-1_e955c : Constant  Value=-1
  Constant_-1_fa595 : Constant  Value=-1
  Constant_-1_fb0e7 : Constant  Value=-1
  Constant_-1_fbda6 : Constant  Value=-1
  Constant_2.0_b168a : Constant  Value=2.0
  Constant_T_qd_fe8f4 : Constant  Value=T_qd
  Constant_x_l_24e30 : Constant  Value=x_l
  Constant_x_l_7baa9 : Constant  Value=x_l
  Constant_x_l_84d36 : Constant  Value=x_l
  Constant_x_l_87845 : Constant  Value=x_l
  Constant_x_l_93664 : Constant  Value=x_l
  Constant_x_l_d447e : Constant  Value=x_l
  Constant_x_l_f8859 : Constant  Value=x_l
  Constant_x_l_fc93a : Constant  Value=x_l
  Constant_x_q_77a08 : Constant  Value=x_q
  Constant_x_qd_23147 : Constant  Value=x_qd
  Constant_x_qd_235c7 : Constant  Value=x_qd
  Constant_x_qd_25c6a : Constant  Value=x_qd
  Constant_x_qd_29108 : Constant  Value=x_qd
  Constant_x_qd_3e223 : Constant  Value=x_qd
  Constant_x_qd_73ba4 : Constant  Value=x_qd
  Constant_x_qd_9cb56 : Constant  Value=x_qd
  Constant_x_qd_cf5a9 : Constant  Value=x_qd
  Constant_x_qd_e23e5 : Constant  Value=x_qd
  Constant_x_qd_fe68a : Constant  Value=x_qd
  Constant_x_qdd_1e168 : Constant  Value=x_qdd
  Constant_x_qdd_716d6 : Constant  Value=x_qdd
  Constant_x_qdd_732b8 : Constant  Value=x_qdd
  Constant_x_qdd_868fd : Constant  Value=x_qdd
  Constant_x_qdd_b705b : Constant  Value=x_qdd
  Constant_x_qdd_dc134 : Constant  Value=x_qdd
  Constant_x_qdd_fa4d3 : Constant  Value=x_qdd
  Divide_1b0b3 : Product  Inputs=*/
  Divide_208d9 : Product  Inputs=*/
  Divide_3a3af : Product  Inputs=*/
  Divide_423fa : Product  Inputs=*/
  Divide_4383c : Product  Inputs=*/
  Divide_63e9f : Product  Inputs=*/
  Divide_6b7aa : Product  Inputs=*/
  Divide_bb130 : Product  Inputs=*/
  Power_1ccc7 : Math  Operator=pow
  Product_19c68 : Product
  Product_1ad2c : Product
  Product_31185 : Product
  Product_36384 : Product
  Product_39d8e : Product
  Product_640dd : Product
  Product_6dad3 : Product
  Product_77bef : Product
  Product_87278 : Product
  Product_ac515 : Product
  Product_ad2b9 : Product
  Product_afa82 : Product
  Product_bbd73 : Product
  Product_d781a : Product
  Product_ddea3 : Product
  Product_e5d30 : Product
  Product_f7beb : Product
  Subtract_01b42 : Sum  Inputs=+-
  Subtract_2f75e : Sum  Inputs=+-
  Subtract_49762 : Sum  Inputs=+-
  Subtract_49dc9 : Sum  Inputs=+-
  Subtract_61104 : Sum  Inputs=+-
  Subtract_8b034 : Sum  Inputs=+-
  Subtract_937f4 : Sum  Inputs=+-
  Subtract_c9687 : Sum  Inputs=+-
  Blockout_d_psi_gq_SG_D_23_82b8d : Outport
  wires:
  Constant_-1_b270e/1 -> Product_d781a/1
  Constant_x_l_84d36/1 -> Product_31185/2
  Constant_-1_e955c/1 -> Product_77bef/1
  Constant_x_l_93664/1 -> Product_d781a/2
  State_psi_kq_SG_D_23_c86ae/1 -> Product_6dad3/1
  Constant_x_l_87845/1 -> Product_1ad2c/2
  Product_d781a/1 -> Add_5d65c/1
  Add_81c60/1 -> Divide_63e9f/2
  Add_6eda3/1 -> Divide_6b7aa/1
  Product_19c68/1 -> Divide_423fa/1
  Constant_x_qdd_868fd/1 -> Add_5d65c/2
  Constant_-1_5ec91/1 -> Product_1ad2c/1
  Constant_x_l_7baa9/1 -> Product_afa82/2
  Constant_x_qd_fe68a/1 -> Subtract_01b42/1
  Constant_x_qdd_732b8/1 -> Subtract_01b42/2
  Constant_x_l_24e30/1 -> Product_f7beb/2
  Constant_-1_74396/1 -> Product_ddea3/1
  Constant_x_l_fc93a/1 -> Product_ddea3/2
  State_psi_gq_SG_D_23_9dcc3/1 -> Product_36384/1
  Constant_x_qdd_716d6/1 -> Add_22213/2
  Add_5d65c/1 -> Product_36384/2
  Constant_x_qdd_b705b/1 -> Subtract_49762/2
  Product_1ad2c/1 -> Add_d9c53/1
  Constant_x_qd_29108/1 -> Add_d9c53/2
  State_psi_gq_SG_D_23_52211/1 -> Add_5c235/1
  Subtract_49762/1 -> Product_6dad3/2
  State_psi_kq_SG_D_23_b4351/1 -> Product_ad2b9/1
  Subtract_01b42/1 -> Product_ad2b9/2
  Product_ddea3/1 -> Add_1b597/1
  Add_22213/1 -> Product_bbd73/2
  Constant_x_qd_25c6a/1 -> Add_1b597/2
  Product_36384/1 -> Divide_3a3af/1
  State_psi_kq_SG_D_23_2d830/1 -> Add_5c235/2
  Add_d9c53/1 -> Divide_3a3af/2
  Product_ad2b9/1 -> Divide_4383c/1
  Add_1b597/1 -> Divide_4383c/2
  Constant_x_qd_73ba4/1 -> Add_81c60/2
  Constant_x_l_f8859/1 -> Product_77bef/2
  Divide_3a3af/1 -> Subtract_49dc9/1
  Divide_4383c/1 -> Subtract_49dc9/2
  Constant_-1_fb0e7/1 -> Product_f7beb/1
  Constant_-1_fbda6/1 -> Product_31185/1
  Product_77bef/1 -> Add_32192/1
  State_psi_q_SG_D_23_a58a4/1 -> Add_ce471/2
  Product_6dad3/1 -> Divide_63e9f/1
  Constant_x_qd_235c7/1 -> Add_32192/2
  Constant_x_qd_cf5a9/1 -> Add_66016/2
  Constant_x_qdd_dc134/1 -> Subtract_61104/2
  Subtract_49dc9/1 -> Add_b1f47/1
  Product_bbd73/1 -> Divide_bb130/1
  State_psi_q_SG_D_23_fd8a2/1 -> Add_b1f47/2
  Product_f7beb/1 -> Add_22213/1
  Constant_-1_d9c78/1 -> Product_87278/1
  Constant_-1_21c54/1 -> Product_e5d30/1
  Add_b1f47/1 -> Product_19c68/2
  Constant_x_l_d447e/1 -> Product_e5d30/2
  Constant_x_qd_9cb56/1 -> Subtract_49762/1
  Product_31185/1 -> Add_81c60/1
  Add_32192/1 -> Product_19c68/1
  Constant_x_qdd_fa4d3/1 -> Divide_423fa/2
  Constant_x_q_77a08/1 -> Subtract_937f4/1
  State_psi_gq_SG_D_23_02c8f/1 -> Product_bbd73/1
  Constant_T_qd_fe8f4/1 -> Divide_6b7aa/2
  Product_e5d30/1 -> Add_66016/1
  Product_640dd/1 -> Add_6eda3/1
  Constant_x_qd_e23e5/1 -> Subtract_61104/1
  Constant_-1_fa595/1 -> Product_afa82/1
  Add_66016/1 -> Divide_bb130/2
  Subtract_61104/1 -> Product_87278/2
  Add_5c235/1 -> Subtract_8b034/1
  Divide_423fa/1 -> Subtract_8b034/2
  Product_afa82/1 -> Add_07245/1
  Constant_x_qd_23147/1 -> Add_07245/2
  Divide_bb130/1 -> Subtract_2f75e/1
  Divide_63e9f/1 -> Subtract_2f75e/2
  Product_87278/1 -> Product_ac515/1
  Subtract_8b034/1 -> Product_ac515/2
  Add_07245/1 -> Power_1ccc7/1
  Constant_2.0_b168a/1 -> Power_1ccc7/2
  Subtract_2f75e/1 -> Add_ce471/1
  Product_ac515/1 -> Divide_208d9/1
  Power_1ccc7/1 -> Divide_208d9/2
  Add_ce471/1 -> Divide_1b0b3/1
  Constant_x_qdd_1e168/1 -> Divide_1b0b3/2
  Constant_x_qd_3e223/1 -> Subtract_937f4/2
  Divide_208d9/1 -> Subtract_c9687/1
  Divide_1b0b3/1 -> Subtract_c9687/2
  Constant_-1_c60a9/1 -> Product_640dd/1
  State_psi_gq_SG_D_23_15800/1 -> Product_640dd/2
  Subtract_937f4/1 -> Product_39d8e/1
  Subtract_c9687/1 -> Product_39d8e/2
  Product_39d8e/1 -> Add_6eda3/2
  Divide_6b7aa/1 -> Blockout_d_psi_gq_SG_D_23_82b8d/1

== system IEEE30_case/SG_D_23/d_psi_kq_SG_D_23_block ==
  note: d_psi_kq_SG_D_23 in IEEE30_case
      | $-\frac{\psi _{\mathrm{gq},\mathrm{SG},D,23}+\psi _{\mathrm{kq},\mathrm{SG},D,23}+\frac{\left(x_{l}-x_{\mathrm{qd}}\right)\,\left(\psi _{q,\mathrm{SG},D,23}+\frac{\psi _{\mathrm{gq},\mathrm{SG},D,23}\,\left(x_{l}-x_{\mathrm{qdd}}\right)}{x_{l}-x_{\mathrm{qd}}}+\frac{\psi _{\mathrm{kq},\mathrm{SG},D,23}\,\left(x_{\mathrm{qd}}-x_{\mathrm{qdd}}\right)}{x_{l}-x_{\mathrm{qd}}}\right)}{x_{\mathrm{qdd}}}}{T_{\mathrm{qdd}}}$
      | Automatically generated on 2025-11-01 18:37:21 .
  State_psi_gq_SG_D_23_ea537 : Inport
  State_psi_kq_SG_D_23_3117e : Inport  Port=2
  State_psi_gq_SG_D_23_bc7a2 : Inport  Port=3
  State_psi_kq_SG_D_23_31b6f : Inport  Port=4
  State_psi_q_SG_D_23_a4607 : Inport  Port=5
  Add_5b483 : Sum
  Add_678b0 : Sum
  Add_7d99d : Sum
  Add_82331 : Sum
  Add_c4f90 : Sum
  Add_d872f : Sum
  Constant_-1_3339d : Constant  Value=-1
  Constant_-1_a2967 : Constant  Value=-1
  Constant_-1_c0476 : Constant  Value=-1
  Constant_-1_d69d0 : Constant  Value=-1
  Constant_-1_d75d5 : Constant  Value=-1
  Constant_T_qdd_22600 : Constant  Value=T_qdd
  Constant_x_l_037a6 : Constant  Value=x_l
  Constant_x_l_38906 : Constant  Value=x_l
  Constant_x_l_6e5c5 : Constant  Value=x_l
  Constant_x_l_8b14e : Constant  Value=x_l
  Constant_x_qd_07660 : Constant  Value=x_qd
  Constant_x_qd_501ac : Constant  Value=x_qd
  Constant_x_qd_d2001 : Constant  Value=x_qd
  Constant_x_qd_fe9c3 : Constant  Value=x_qd
  Constant_x_qdd_1761f : Constant  Value=x_qdd
  Constant_x_qdd_46aa5 : Constant  Value=x_qdd
  Constant_x_qdd_5a3a5 : Constant  Value=x_qdd
  Divide_2cd5e : Product  Inputs=*/
  Divide_402e2 : Product  Inputs=*/
  Divide_af15e : Product  Inputs=*/
  Divide_cfa36 : Product  Inputs=*/
  Product_012c9 : Product
  Product_3de57 : Product
  Product_80cfc : Product
  Product_8e32e : Product
  Product_c2b82 : Product
  Product_d1dc2 : Product
  Product_d9609 : Product
  Product_e1a0b : Product
  Subtract_4c182 : Sum  Inputs=+-
  Subtract_7e107 : Sum  Inputs=+-
  Subtract_d6f95 : Sum  Inputs=+-
  Blockout_d_psi_kq_SG_D_23_e5927 : Outport
  wires:
  Constant_-1_c0476/1 -> Product_d9609/1
  Constant_x_qd_fe9c3/1 -> Add_d872f/2
  Constant_x_l_037a6/1 -> Product_d9609/2
  Product_d9609/1 -> Add_82331/1
  Constant_x_l_38906/1 -> Product_012c9/2
  Constant_x_qdd_1761f/1 -> Add_82331/2
  Constant_-1_3339d/1 -> Product_012c9/1
  Constant_-1_d75d5/1 -> Product_e1a0b/1
  Constant_x_qd_07660/1 -> Subtract_7e107/1
  Constant_x_qdd_5a3a5/1 -> Subtract_7e107/2
  Constant_-1_d69d0/1 -> Product_80cfc/1
  Constant_x_l_8b14e/1 -> Product_80cfc/2
  State_psi_gq_SG_D_23_bc7a2/1 -> Product_8e32e/1
  Add_82331/1 -> Product_8e32e/2
  Product_012c9/1 -> Add_5b483/1
  Constant_x_qdd_46aa5/1 -> Divide_402e2/2
  Subtract_4c182/1 -> Add_678b0/1
  Constant_x_qd_d2001/1 -> Add_5b483/2
  State_psi_kq_SG_D_23_31b6f/1 -> Product_3de57/1
  Subtract_7e107/1 -> Product_3de57/2
  Product_80cfc/1 -> Add_d872f/1
  Product_8e32e/1 -> Divide_af15e/1
  Add_5b483/1 -> Divide_af15e/2
  Constant_-1_a2967/1 -> Product_d1dc2/1
  Product_3de57/1 -> Divide_2cd5e/1
  Divide_cfa36/1 -> Blockout_d_psi_kq_SG_D_23_e5927/1
  State_psi_kq_SG_D_23_3117e/1 -> Subtract_d6f95/2
  Add_d872f/1 -> Divide_2cd5e/2
  Constant_x_l_6e5c5/1 -> Product_e1a0b/2
  Divide_af15e/1 -> Subtract_4c182/1
  Product_d1dc2/1 -> Subtract_d6f95/1
  Divide_2cd5e/1 -> Subtract_4c182/2
  Product_e1a0b/1 -> Add_c4f90/1
  Constant_x_qd_501ac/1 -> Add_c4f90/2
  State_psi_q_SG_D_23_a4607/1 -> Add_678b0/2
  State_psi_gq_SG_D_23_ea537/1 -> Product_d1dc2/2
  Add_c4f90/1 -> Product_c2b82/1
  Add_678b0/1 -> Product_c2b82/2
  Product_c2b82/1 -> Divide_402e2/1
  Subtract_d6f95/1 -> Add_7d99d/1
  Divide_402e2/1 -> Add_7d99d/2
  Add_7d99d/1 -> Divide_cfa36/1
  Constant_T_qdd_22600/1 -> Divide_cfa36/2

== system IEEE30_case/SG_D_23/d_psi_q_SG_D_23_block ==
  note: d_psi_q_SG_D_23 in IEEE30_case
      | $2\,\pi \,f_{0}\,\left(v_{d,\mathrm{SG},D,23}\,\cos\left(\theta _{\mathrm{SG},D,23}\right)+v_{q,\mathrm{SG},D,23}\,\sin\left(\theta _{\mathrm{SG},D,23}\right)-\frac{R_{a}\,\left(\psi _{q,\mathrm{SG},D,23}+\frac{\psi _{\mathrm{gq},\mathrm{SG},D,23}\,\left(x_{l}-x_{\mathrm{qdd}}\right)}{x_{l}-x_{\mathrm{qd}}}+\frac{\psi _{\mathrm{kq},\mathrm{SG},D,23}\,\left(x_{\mathrm{qd}}-x_{\mathrm{qdd}}\right)}{x_{l}-x_{\mathrm{qd}}}\right)}{x_{\mathrm{qdd}}}-\frac{\psi _{d,\mathrm{SG},D,23}\,w_{\mathrm{SG},D,23}}{2\,f_{0}\,\pi }\right)$
      | Automatically generated on 2025-11-01 18:37:03 .
  State_psi_gq_SG_D_23_36696 : Inport
  State_psi_kq_SG_D_23_a5d65 : Inport  Port=2
  State_psi_q_SG_D_23_cf2f8 : Inport  Port=3
  Input_v_d_SG_D_23_a1330 : Inport  Port=4
  State_theta_SG_D_23_d0e02 : Inport  Port=5
  Input_v_q_SG_D_23_6ddda : Inport  Port=6
  State_theta_SG_D_23_99733 : Inport  Port=7
  State_psi_d_SG_D_23_d98d6 : Inport  Port=8
  State_w_SG_D_23_ea7ff : Inport  Port=9
  Add_068b6 : Sum
  Add_31215 : Sum
  Add_5967f : Sum
  Add_b298a : Sum
  Add_e1a91 : Sum
  Constant_-1_28bcb : Constant  Value=-1
  Constant_-1_2e054 : Constant  Value=-1
  Constant_-1_781ac : Constant  Value=-1
  Constant_-2.0_78ec4 : Constant  Value=-2.0
  Constant_2.0_6a56f : Constant  Value=2.0
  Constant_R_a_c8edf : Constant  Value=R_a
  Constant_f0_3ac6e : Constant  Value=f0
  Constant_f0_6e667 : Constant  Value=f0
  Constant_pi_8b376 : Constant  Value=pi
  Constant_pi_bb07b : Constant  Value=pi
  Constant_x_l_1a661 : Constant  Value=x_l
  Constant_x_l_21d31 : Constant  Value=x_l
  Constant_x_l_a778d : Constant  Value=x_l
  Constant_x_qd_0dbd1 : Constant  Value=x_qd
  Constant_x_qd_6941c : Constant  Value=x_qd
  Constant_x_qd_7691d : Constant  Value=x_qd
  Constant_x_qdd_27bb6 : Constant  Value=x_qdd
  Constant_x_qdd_8d890 : Constant  Value=x_qdd
  Constant_x_qdd_c94ff : Constant  Value=x_qdd
  Divide_63237 : Product  Inputs=*/
  Divide_88611 : Product  Inputs=*/
  Divide_cfce9 : Product  Inputs=*/
  Divide_de726 : Product  Inputs=*/
  MathFunc_cos_0ca80 : Trigonometry  Operator=cos
  MathFunc_sin_5d3df : Trigonometry
  Product_1a402 : Product
  Product_1a48e : Product
  Product_1fd38 : Product
  Product_23a0b : Product
  Product_3084d : Product
  Product_30b71 : Product
  Product_34699 : Product
  Product_4ae9f : Product
  Product_4cf06 : Product
  Product_9637c : Product
  Product_c89f6 : Product
  Product_cbc89 : Product
  Product_d9761 : Product
  Product_fe428 : Product
  Subtract_3759d : Sum  Inputs=+-
  Subtract_f0dc0 : Sum  Inputs=+-
  Subtract_f1c09 : Sum  Inputs=+-
  Subtract_f8eee : Sum  Inputs=+-
  Blockout_d_psi_q_SG_D_23_cbd1d : Outport
  wires:
  Constant_f0_6e667/1 -> Product_3084d/2
  Constant_x_l_1a661/1 -> Product_1fd38/2
  Constant_-1_28bcb/1 -> Product_34699/1
  Product_34699/1 -> Add_e1a91/1
  Subtract_f0dc0/1 -> Subtract_3759d/1
  Constant_x_l_a778d/1 -> Product_34699/2
  Subtract_f8eee/1 -> Add_5967f/1
  Constant_x_qd_0dbd1/1 -> Subtract_f1c09/1
  Constant_x_qdd_27bb6/1 -> Add_e1a91/2
  Divide_cfce9/1 -> Subtract_f0dc0/1
  Constant_-1_781ac/1 -> Product_1fd38/1
  Divide_88611/1 -> Subtract_f8eee/1
  Constant_x_qdd_c94ff/1 -> Subtract_f1c09/2
  Product_1a402/1 -> Blockout_d_psi_q_SG_D_23_cbd1d/1
  Constant_pi_bb07b/1 -> Product_fe428/2
  Product_cbc89/1 -> Divide_cfce9/1
  Constant_-1_2e054/1 -> Product_30b71/1
  Constant_x_l_21d31/1 -> Product_30b71/2
  Add_068b6/1 -> Product_1a402/2
  Subtract_3759d/1 -> Add_068b6/1
  State_psi_gq_SG_D_23_36696/1 -> Product_1a48e/1
  Add_e1a91/1 -> Product_1a48e/2
  Product_1fd38/1 -> Add_b298a/1
  Constant_x_qd_7691d/1 -> Add_b298a/2
  State_psi_kq_SG_D_23_a5d65/1 -> Product_4ae9f/1
  Subtract_f1c09/1 -> Product_4ae9f/2
  Product_30b71/1 -> Add_31215/1
  Product_fe428/1 -> Product_c89f6/1
  Constant_x_qd_6941c/1 -> Add_31215/2
  Product_1a48e/1 -> Divide_88611/1
  Add_b298a/1 -> Divide_88611/2
  Product_4ae9f/1 -> Divide_de726/1
  Add_31215/1 -> Divide_de726/2
  Divide_de726/1 -> Subtract_f8eee/2
  Constant_2.0_6a56f/1 -> Product_fe428/1
  State_psi_q_SG_D_23_cf2f8/1 -> Add_5967f/2
  Product_3084d/1 -> Product_1a402/1
  Divide_63237/1 -> Add_068b6/2
  Constant_R_a_c8edf/1 -> Product_cbc89/1
  Add_5967f/1 -> Product_cbc89/2
  MathFunc_cos_0ca80/1 -> Product_4cf06/2
  State_theta_SG_D_23_d0e02/1 -> MathFunc_cos_0ca80/1
  Product_c89f6/1 -> Divide_63237/2
  Constant_x_qdd_8d890/1 -> Divide_cfce9/2
  Input_v_d_SG_D_23_a1330/1 -> Product_4cf06/1
  State_theta_SG_D_23_99733/1 -> MathFunc_sin_5d3df/1
  Product_4cf06/1 -> Subtract_f0dc0/2
  Product_d9761/1 -> Subtract_3759d/2
  Input_v_q_SG_D_23_6ddda/1 -> Product_d9761/1
  MathFunc_sin_5d3df/1 -> Product_d9761/2
  State_psi_d_SG_D_23_d98d6/1 -> Product_23a0b/1
  State_w_SG_D_23_ea7ff/1 -> Product_23a0b/2
  Constant_f0_3ac6e/1 -> Product_c89f6/2
  Constant_-2.0_78ec4/1 -> Product_9637c/1
  Constant_pi_8b376/1 -> Product_9637c/2
  Product_9637c/1 -> Product_3084d/1
  Product_23a0b/1 -> Divide_63237/1

== system IEEE30_case/SG_D_23/d_theta_SG_D_23_block ==
  note: d_theta_SG_D_23 in IEEE30_case
      | $w_{\mathrm{SG},D,23}-2\,\pi \,f_{0}$
      | Automatically generated on 2025-11-01 18:37:28 .
  State_w_SG_D_23_9ae8c : Inport
  Add_262b7 : Sum
  Constant_-2.0_72527 : Constant  Value=-2.0
  Constant_f0_ab14b : Constant  Value=f0
  Constant_pi_113c7 : Constant  Value=pi
  Product_90cfc : Product
  Product_ec33a : Product
  Blockout_d_theta_SG_D_23_51717 : Outport
  wires:
  Constant_-2.0_72527/1 -> Product_90cfc/1
  Product_ec33a/1 -> Add_262b7/1
  Constant_pi_113c7/1 -> Product_90cfc/2
  Product_90cfc/1 -> Product_ec33a/1
  State_w_SG_D_23_9ae8c/1 -> Add_262b7/2
  Constant_f0_ab14b/1 -> Product_ec33a/2
  Add_262b7/1 -> Blockout_d_theta_SG_D_23_51717/1
